simulink model "Eq2_SOC_VOC"  (R2022b)
settings: Solver=FixedStepAuto  StartTime=0.0  StopTime=10.0  RelTol=1e-3
settings Model: Creator=umber  LastModifiedBy=umber
settings OptimizationCC: OptimizeBlockIOStorage=off  OptimizeDataStoreBuffers=off  BusAssignmentInplaceUpdate=off
settings DebuggingCC: SFUnexpectedBacktrackingDiag=warning  SFNoUnconditionalDefaultTransitionDiag=warning
settings ModelReferenceCC: EnableRefExpFcnMdlSchedulingChecks=on
settings RTWCC: GenCodeOnly=on  GenerateReport=on  BuildConfiguration=Debug  LaunchReport=on
settings CodeAppCC: ForceParamTrailComments=on  MATLABSourceComments=on  EnableCustomComments=on
settings GRTTargetCC: CombineSignalStateStructs=on  SupportVariableSizeSignals=on  MultiInstanceErrorCode=Warning

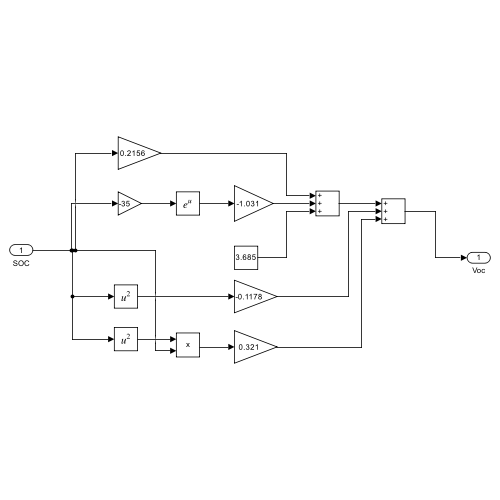
[thumbnail: Simulink's stored preview of the top-level diagram]
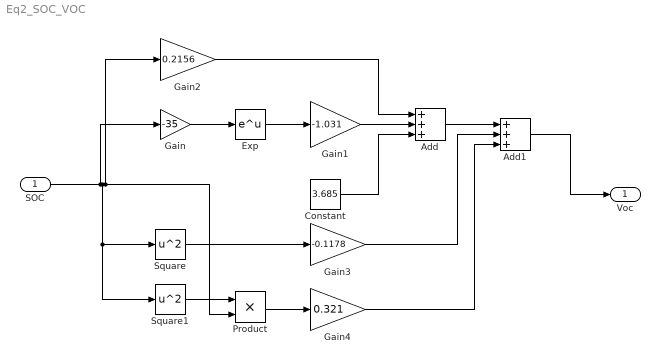
== system Eq2_SOC_VOC ==
  SOC : Inport
  Add : Sum  Inputs=+++
  Add1 : Sum  Inputs=+++
  Constant : Constant  Value=3.685
  Exp : Math
  Gain : Gain  Gain=-35
  Gain1 : Gain  Gain=-1.031
  Gain2 : Gain  Gain=0.2156
  Gain3 : Gain  Gain=-0.1178
  Gain4 : Gain  Gain=0.321
  Product : Product
  Square : Math  Operator=square
  Square1 : Math  Operator=square
  Voc : Outport
  wires:
  Add1/1 -> Voc/1
  Gain3/1 -> Add1/2
  Constant/1 -> Add/3
  Square/1 -> Gain3/1
  Square1/1 -> Product/1
  Gain4/1 -> Add1/3
  Product/1 -> Gain4/1
  Add/1 -> Add1/1
  Gain/1 -> Exp/1
  Gain1/1 -> Add/2
  Gain2/1 -> Add/1
  Exp/1 -> Gain1/1
  SOC/1 -> Square1/1, Square/1, Product/2, Gain2/1, Gain/1
